simulink model "TCLab_heaterSliders_test"  (R2022b)
settings: Solver=FixedStepAuto  StartTime=0.0  StopTime=300  RelTol=1e-3  EnableMultiTasking=on
libraries: arduinolib x5
settings Model: ExtModeTrigDuration=2  Creator=samvithr  LastModifiedBy=Afonso
settings SolverCC: AlgebraicLoopSolver=TrustRegion
settings OptimizationCC: EnhancedBackFolding=on  PassReuseOutputArgsThreshold=0  MaxStackSize=64  OptimizeBlockOrder=speed  DifferentSizesBufferReuse=on  OptimizationCustomize=off
settings DebuggingCC: ParameterTunabilityLossMsg=error  UnconnectedInputMsg=warning  UnconnectedOutputMsg=warning  UnconnectedLineMsg=warning  SFMachineParentedDataDiag=warning
settings HardwareCC: ProdBitPerInt=16  ProdBitPerPointer=16  ProdBitPerSizeT=16  ProdBitPerPtrDiffT=16  ProdLargestAtomicFloat=None  ProdWordSize=8  ProdHWDeviceType=Atmel->AVR
settings ModelReferenceCC: EnableRefExpFcnMdlSchedulingChecks=on
settings SFSimCC: MATLABDynamicMemAlloc=off  CustomCodeUndefinedFunction=UseInterfaceOnly
settings RTWCC: Description=Embedded Coder  SystemTargetFile=ert.tlc  HardwareBoard=Arduino Leonardo  TLCOptions=-aInlineSetEventsForThisBaseRateFcn=TLC_FALSE -aSuppressMultiTaskScheduler=TLC_FALSE -aRateBasedStepFcn=1  TemplateMakefile=ert_default_tmf  GenerateReport=on  Toolchain=Arduino AVR  BuildConfiguration=Faster Runs  LaunchReport=on
settings CodeAppCC: ForceParamTrailComments=on  OperatorAnnotations=on
settings ERTTargetCC: ERTCustomFileBanners=off  SupportContinuousTime=on  SupportNonInlinedSFcns=on  RemoveResetFunc=off  SupportVariableSizeSignals=on  ModelStepFunctionPrototypeControlCompliant=off  ExtModeTransport=3  ExtModeStaticAlloc=on  ExtModeAutomaticAllocSize=off  ExtModeStaticAllocSize=250  ExtModeMexFile=ext_xcp  ExtModeIntrfLevel=Level2 - Open

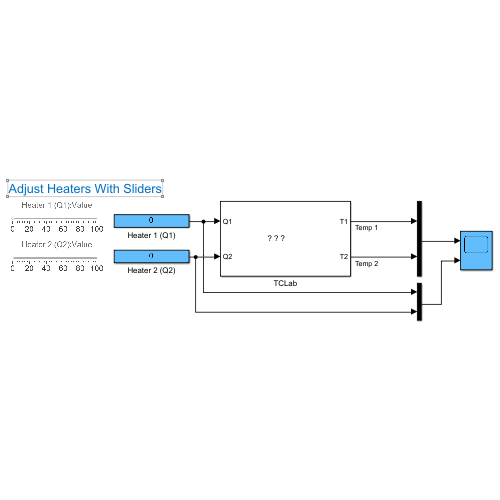
[thumbnail: Simulink's stored preview of the top-level diagram]
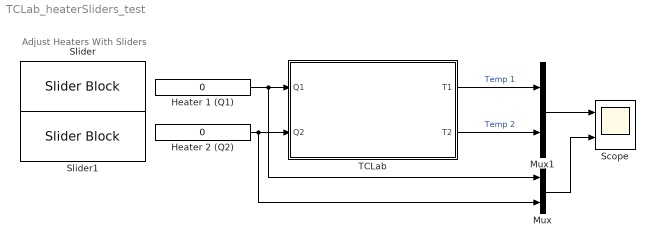
== system TCLab_heaterSliders_test ==
  note: Adjust Heaters With Sliders
  Heater 1 (Q1) : Constant  Value=0
  Heater 2 (Q2) : Constant  Value=0
  Mux : Mux  Inputs=2
  Mux1 : Mux  Inputs=2
  Scope : Scope  NumInputPorts=2
  Slider : SliderBlock  TickInterval=20
  Slider1 : SliderBlock  TickInterval=20
  TCLab : Subsystem
      mask Display: image('Arduino.png');
  wires:
  Heater 2 (Q2)/1 -> Mux/2, TCLab/2(Q2)
  Heater 1 (Q1)/1 -> Mux/1, TCLab/1(Q1)
  TCLab/1(T1) -> Mux1/1  "Temp 1"
  TCLab/2(T2) -> Mux1/2  "Temp 2"
  Mux1/1 -> Scope/1
  Mux/1 -> Scope/2

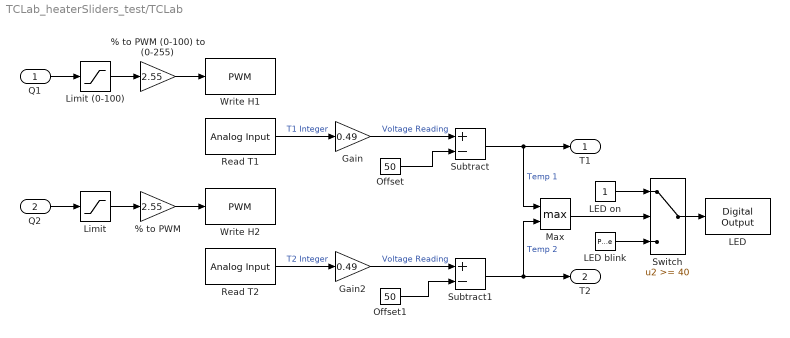
== system TCLab_heaterSliders_test/TCLab ==
  Q1 : Inport
  Q2 : Inport  Port=2
  % to PWM (0-100) to (0-255) : Gain  Gain=2.55
  "% to PWM " : Gain  Gain=2.55
  Gain : Gain  Gain=0.49
  Gain2 : Gain  Gain=0.49
  LED : arduinolib/Digital Output  pinNumber=9  Direction=output  blockPlatform=arduino
  LED blink : DiscretePulseGenerator  Period=4  PulseWidth=2  SampleTime=0.5
  LED on : Constant
  Limit : Saturate  UpperLimit=100  LowerLimit=0
  Limit (0-100) : Saturate  UpperLimit=100  LowerLimit=0
  Max : MinMax  Function=max  Inputs=2
  Offset : Constant  Value=50
  Offset1 : Constant  Value=50
  Read T1 : arduinolib/Analog Input  pinNumber=0  ReadResultsOnly=off  ConversionTriggerSource=Software  ExternalTriggerType=uint32(0)  OutputDataType=uint16  EnableConversionCompleteNotify=off  EnableOuputStatus=off  SampleTime=0.5  blockPlatform=arduino
  Read T2 : arduinolib/Analog Input  pinNumber=2  ReadResultsOnly=off  ConversionTriggerSource=Software  ExternalTriggerType=uint32(0)  OutputDataType=uint16  EnableConversionCompleteNotify=off  EnableOuputStatus=off  SampleTime=0.5  blockPlatform=arduino
  Subtract : Sum  Inputs=+-
  Subtract1 : Sum  Inputs=+-
  Switch : Switch  Threshold=40  SaturateOnIntegerOverflow=off  InputSameDT=off
  Write H1 : arduinolib/PWM  pinNumber=3  frequencyType=Default  desiredFrequency=490.2  achievableFrequency=490.2
  Write H2 : arduinolib/PWM  pinNumber=5  frequencyType=Default  desiredFrequency=490.2  achievableFrequency=490.2
  T1 : Outport  VectorParamsAs1DForOutWhenUnconnected=off
  T2 : Outport  Port=2  VectorParamsAs1DForOutWhenUnconnected=off
  wires:
  Gain/1 -> Subtract/1  "Voltage Reading"
  Offset/1 -> Subtract/2
  Read T1/1 -> Gain/1  "T1 Integer"
  Subtract/1 -> Max/1, T1/1  "Temp 1"
  Limit (0-100)/1 -> % to PWM (0-100) to (0-255)/1
  % to PWM (0-100) to (0-255)/1 -> Write H1/1
  Switch/1 -> LED/1
  LED on/1 -> Switch/1
  LED blink/1 -> Switch/3
  Read T2/1 -> Gain2/1  "T2 Integer"
  Subtract1/1 -> Max/2, T2/1  "Temp 2"
  Gain2/1 -> Subtract1/1  "Voltage Reading"
  "% to PWM "/1 -> Write H2/1
  Offset1/1 -> Subtract1/2
  Max/1 -> Switch/2
  Q1/1 -> Limit (0-100)/1
  Q2/1 -> Limit/1
  Limit/1 -> "% to PWM "/1
